simulink model "c00006M_harness"  (R2018a)
settings: Solver=FixedStepAuto  StartTime=0.0  StopTime=300  FixedStep=0.1  RelTol=1e-3
undefined symbols (not defined in the file): A1, hmax, PriorityTank, R1, R2, sigbuilder_block, TempThreshold
(part 3 of 66)

== system c00006M_harness/Eval150 ==
  In2 : Inport
  In3 : Inport  Port=2
  Constant1 : Constant
  Data Type Conversion1 : DataTypeConversion
  Data Type Conversion2 : DataTypeConversion
  Memory2 : Memory  InitialCondition=1
  Memory3 : Memory  InitialCondition=1
  MinMax : MinMax  Inputs=3
  MinMax2 : MinMax  Inputs=2
  MinMax3 : MinMax  Inputs=2
  ROOut2 : RelationalOperator  Operator===  OutDataTypeStr=boolean  RndMeth=Simplest
  ROOut3 : RelationalOperator  Operator===  OutDataTypeStr=boolean  RndMeth=Simplest
  Out1 : Outport
  wires:
  Data Type Conversion2/1 -> MinMax3/1
  Data Type Conversion1/1 -> MinMax2/1
  MinMax2/1 -> MinMax/2, Memory2/1
  Memory2/1 -> MinMax2/2
  Memory3/1 -> MinMax3/2
  ROOut2/1 -> Data Type Conversion1/1
  ROOut3/1 -> Data Type Conversion2/1
  MinMax3/1 -> Memory3/1, MinMax/3
  [out2] -> ROOut2/2
  In2/1 -> ROOut2/1
  In3/1 -> ROOut3/1
  [out3] -> ROOut3/2
  MinMax/1 -> Out1/1
  Constant1/1 -> MinMax/1

== system c00006M_harness/Eval151 ==
  In2 : Inport
  In3 : Inport  Port=2
  Constant1 : Constant
  Data Type Conversion1 : DataTypeConversion
  Data Type Conversion2 : DataTypeConversion
  Memory2 : Memory  InitialCondition=1
  Memory3 : Memory  InitialCondition=1
  MinMax : MinMax  Inputs=3
  MinMax2 : MinMax  Inputs=2
  MinMax3 : MinMax  Inputs=2
  ROOut2 : RelationalOperator  Operator===  OutDataTypeStr=boolean  RndMeth=Simplest
  ROOut3 : RelationalOperator  Operator===  OutDataTypeStr=boolean  RndMeth=Simplest
  Out1 : Outport
  wires:
  Data Type Conversion2/1 -> MinMax3/1
  Data Type Conversion1/1 -> MinMax2/1
  MinMax2/1 -> MinMax/2, Memory2/1
  Memory2/1 -> MinMax2/2
  Memory3/1 -> MinMax3/2
  ROOut2/1 -> Data Type Conversion1/1
  ROOut3/1 -> Data Type Conversion2/1
  MinMax3/1 -> Memory3/1, MinMax/3
  [out2] -> ROOut2/2
  In2/1 -> ROOut2/1
  In3/1 -> ROOut3/1
  [out3] -> ROOut3/2
  MinMax/1 -> Out1/1
  Constant1/1 -> MinMax/1

== system c00006M_harness/Eval152 ==
  In2 : Inport
  In3 : Inport  Port=2
  Constant1 : Constant
  Data Type Conversion1 : DataTypeConversion
  Data Type Conversion2 : DataTypeConversion
  Memory2 : Memory  InitialCondition=1
  Memory3 : Memory  InitialCondition=1
  MinMax : MinMax  Inputs=3
  MinMax2 : MinMax  Inputs=2
  MinMax3 : MinMax  Inputs=2
  ROOut2 : RelationalOperator  Operator===  OutDataTypeStr=boolean  RndMeth=Simplest
  ROOut3 : RelationalOperator  Operator===  OutDataTypeStr=boolean  RndMeth=Simplest
  Out1 : Outport
  wires:
  Data Type Conversion2/1 -> MinMax3/1
  Data Type Conversion1/1 -> MinMax2/1
  MinMax2/1 -> MinMax/2, Memory2/1
  Memory2/1 -> MinMax2/2
  Memory3/1 -> MinMax3/2
  ROOut2/1 -> Data Type Conversion1/1
  ROOut3/1 -> Data Type Conversion2/1
  MinMax3/1 -> Memory3/1, MinMax/3
  [out2] -> ROOut2/2
  In2/1 -> ROOut2/1
  In3/1 -> ROOut3/1
  [out3] -> ROOut3/2
  MinMax/1 -> Out1/1
  Constant1/1 -> MinMax/1

== system c00006M_harness/Eval153 ==
  In2 : Inport
  In3 : Inport  Port=2
  Constant1 : Constant
  Data Type Conversion1 : DataTypeConversion
  Data Type Conversion2 : DataTypeConversion
  Memory2 : Memory  InitialCondition=1
  Memory3 : Memory  InitialCondition=1
  MinMax : MinMax  Inputs=3
  MinMax2 : MinMax  Inputs=2
  MinMax3 : MinMax  Inputs=2
  ROOut2 : RelationalOperator  Operator===  OutDataTypeStr=boolean  RndMeth=Simplest
  ROOut3 : RelationalOperator  Operator===  OutDataTypeStr=boolean  RndMeth=Simplest
  Out1 : Outport
  wires:
  Data Type Conversion2/1 -> MinMax3/1
  Data Type Conversion1/1 -> MinMax2/1
  MinMax2/1 -> MinMax/2, Memory2/1
  Memory2/1 -> MinMax2/2
  Memory3/1 -> MinMax3/2
  ROOut2/1 -> Data Type Conversion1/1
  ROOut3/1 -> Data Type Conversion2/1
  MinMax3/1 -> Memory3/1, MinMax/3
  [out2] -> ROOut2/2
  In2/1 -> ROOut2/1
  In3/1 -> ROOut3/1
  [out3] -> ROOut3/2
  MinMax/1 -> Out1/1
  Constant1/1 -> MinMax/1

== system c00006M_harness/Eval154 ==
  In2 : Inport
  In3 : Inport  Port=2
  Constant1 : Constant
  Data Type Conversion1 : DataTypeConversion
  Data Type Conversion2 : DataTypeConversion
  Memory2 : Memory  InitialCondition=1
  Memory3 : Memory  InitialCondition=1
  MinMax : MinMax  Inputs=3
  MinMax2 : MinMax  Inputs=2
  MinMax3 : MinMax  Inputs=2
  ROOut2 : RelationalOperator  Operator===  OutDataTypeStr=boolean  RndMeth=Simplest
  ROOut3 : RelationalOperator  Operator===  OutDataTypeStr=boolean  RndMeth=Simplest
  Out1 : Outport
  wires:
  Data Type Conversion2/1 -> MinMax3/1
  Data Type Conversion1/1 -> MinMax2/1
  MinMax2/1 -> MinMax/2, Memory2/1
  Memory2/1 -> MinMax2/2
  Memory3/1 -> MinMax3/2
  ROOut2/1 -> Data Type Conversion1/1
  ROOut3/1 -> Data Type Conversion2/1
  MinMax3/1 -> Memory3/1, MinMax/3
  [out2] -> ROOut2/2
  In2/1 -> ROOut2/1
  In3/1 -> ROOut3/1
  [out3] -> ROOut3/2
  MinMax/1 -> Out1/1
  Constant1/1 -> MinMax/1

== system c00006M_harness/Eval155 ==
  In2 : Inport
  In3 : Inport  Port=2
  Constant1 : Constant
  Data Type Conversion1 : DataTypeConversion
  Data Type Conversion2 : DataTypeConversion
  Memory2 : Memory  InitialCondition=1
  Memory3 : Memory  InitialCondition=1
  MinMax : MinMax  Inputs=3
  MinMax2 : MinMax  Inputs=2
  MinMax3 : MinMax  Inputs=2
  ROOut2 : RelationalOperator  Operator===  OutDataTypeStr=boolean  RndMeth=Simplest
  ROOut3 : RelationalOperator  Operator===  OutDataTypeStr=boolean  RndMeth=Simplest
  Out1 : Outport
  wires:
  Data Type Conversion2/1 -> MinMax3/1
  Data Type Conversion1/1 -> MinMax2/1
  MinMax2/1 -> MinMax/2, Memory2/1
  Memory2/1 -> MinMax2/2
  Memory3/1 -> MinMax3/2
  ROOut2/1 -> Data Type Conversion1/1
  ROOut3/1 -> Data Type Conversion2/1
  MinMax3/1 -> Memory3/1, MinMax/3
  [out2] -> ROOut2/2
  In2/1 -> ROOut2/1
  In3/1 -> ROOut3/1
  [out3] -> ROOut3/2
  MinMax/1 -> Out1/1
  Constant1/1 -> MinMax/1

== system c00006M_harness/Eval156 ==
  In2 : Inport
  In3 : Inport  Port=2
  Constant1 : Constant
  Data Type Conversion1 : DataTypeConversion
  Data Type Conversion2 : DataTypeConversion
  Memory2 : Memory  InitialCondition=1
  Memory3 : Memory  InitialCondition=1
  MinMax : MinMax  Inputs=3
  MinMax2 : MinMax  Inputs=2
  MinMax3 : MinMax  Inputs=2
  ROOut2 : RelationalOperator  Operator===  OutDataTypeStr=boolean  RndMeth=Simplest
  ROOut3 : RelationalOperator  Operator===  OutDataTypeStr=boolean  RndMeth=Simplest
  Out1 : Outport
  wires:
  Data Type Conversion2/1 -> MinMax3/1
  Data Type Conversion1/1 -> MinMax2/1
  MinMax2/1 -> MinMax/2, Memory2/1
  Memory2/1 -> MinMax2/2
  Memory3/1 -> MinMax3/2
  ROOut2/1 -> Data Type Conversion1/1
  ROOut3/1 -> Data Type Conversion2/1
  MinMax3/1 -> Memory3/1, MinMax/3
  [out2] -> ROOut2/2
  In2/1 -> ROOut2/1
  In3/1 -> ROOut3/1
  [out3] -> ROOut3/2
  MinMax/1 -> Out1/1
  Constant1/1 -> MinMax/1

== system c00006M_harness/Eval157 ==
  In2 : Inport
  In3 : Inport  Port=2
  Constant1 : Constant
  Data Type Conversion1 : DataTypeConversion
  Data Type Conversion2 : DataTypeConversion
  Memory2 : Memory  InitialCondition=1
  Memory3 : Memory  InitialCondition=1
  MinMax : MinMax  Inputs=3
  MinMax2 : MinMax  Inputs=2
  MinMax3 : MinMax  Inputs=2
  ROOut2 : RelationalOperator  Operator===  OutDataTypeStr=boolean  RndMeth=Simplest
  ROOut3 : RelationalOperator  Operator===  OutDataTypeStr=boolean  RndMeth=Simplest
  Out1 : Outport
  wires:
  Data Type Conversion2/1 -> MinMax3/1
  Data Type Conversion1/1 -> MinMax2/1
  MinMax2/1 -> MinMax/2, Memory2/1
  Memory2/1 -> MinMax2/2
  Memory3/1 -> MinMax3/2
  ROOut2/1 -> Data Type Conversion1/1
  ROOut3/1 -> Data Type Conversion2/1
  MinMax3/1 -> Memory3/1, MinMax/3
  [out2] -> ROOut2/2
  In2/1 -> ROOut2/1
  In3/1 -> ROOut3/1
  [out3] -> ROOut3/2
  MinMax/1 -> Out1/1
  Constant1/1 -> MinMax/1

== system c00006M_harness/Eval158 ==
  In2 : Inport
  In3 : Inport  Port=2
  Constant1 : Constant
  Data Type Conversion1 : DataTypeConversion
  Data Type Conversion2 : DataTypeConversion
  Memory2 : Memory  InitialCondition=1
  Memory3 : Memory  InitialCondition=1
  MinMax : MinMax  Inputs=3
  MinMax2 : MinMax  Inputs=2
  MinMax3 : MinMax  Inputs=2
  ROOut2 : RelationalOperator  Operator===  OutDataTypeStr=boolean  RndMeth=Simplest
  ROOut3 : RelationalOperator  Operator===  OutDataTypeStr=boolean  RndMeth=Simplest
  Out1 : Outport
  wires:
  Data Type Conversion2/1 -> MinMax3/1
  Data Type Conversion1/1 -> MinMax2/1
  MinMax2/1 -> MinMax/2, Memory2/1
  Memory2/1 -> MinMax2/2
  Memory3/1 -> MinMax3/2
  ROOut2/1 -> Data Type Conversion1/1
  ROOut3/1 -> Data Type Conversion2/1
  MinMax3/1 -> Memory3/1, MinMax/3
  [out2] -> ROOut2/2
  In2/1 -> ROOut2/1
  In3/1 -> ROOut3/1
  [out3] -> ROOut3/2
  MinMax/1 -> Out1/1
  Constant1/1 -> MinMax/1

== system c00006M_harness/Eval159 ==
  In2 : Inport
  In3 : Inport  Port=2
  Constant1 : Constant
  Data Type Conversion1 : DataTypeConversion
  Data Type Conversion2 : DataTypeConversion
  Memory2 : Memory  InitialCondition=1
  Memory3 : Memory  InitialCondition=1
  MinMax : MinMax  Inputs=3
  MinMax2 : MinMax  Inputs=2
  MinMax3 : MinMax  Inputs=2
  ROOut2 : RelationalOperator  Operator===  OutDataTypeStr=boolean  RndMeth=Simplest
  ROOut3 : RelationalOperator  Operator===  OutDataTypeStr=boolean  RndMeth=Simplest
  Out1 : Outport
  wires:
  Data Type Conversion2/1 -> MinMax3/1
  Data Type Conversion1/1 -> MinMax2/1
  MinMax2/1 -> MinMax/2, Memory2/1
  Memory2/1 -> MinMax2/2
  Memory3/1 -> MinMax3/2
  ROOut2/1 -> Data Type Conversion1/1
  ROOut3/1 -> Data Type Conversion2/1
  MinMax3/1 -> Memory3/1, MinMax/3
  [out2] -> ROOut2/2
  In2/1 -> ROOut2/1
  In3/1 -> ROOut3/1
  [out3] -> ROOut3/2
  MinMax/1 -> Out1/1
  Constant1/1 -> MinMax/1

== system c00006M_harness/Eval160 ==
  In2 : Inport
  In3 : Inport  Port=2
  Constant1 : Constant
  Data Type Conversion1 : DataTypeConversion
  Data Type Conversion2 : DataTypeConversion
  Memory2 : Memory  InitialCondition=1
  Memory3 : Memory  InitialCondition=1
  MinMax : MinMax  Inputs=3
  MinMax2 : MinMax  Inputs=2
  MinMax3 : MinMax  Inputs=2
  ROOut2 : RelationalOperator  Operator===  OutDataTypeStr=boolean  RndMeth=Simplest
  ROOut3 : RelationalOperator  Operator===  OutDataTypeStr=boolean  RndMeth=Simplest
  Out1 : Outport
  wires:
  Data Type Conversion2/1 -> MinMax3/1
  Data Type Conversion1/1 -> MinMax2/1
  MinMax2/1 -> MinMax/2, Memory2/1
  Memory2/1 -> MinMax2/2
  Memory3/1 -> MinMax3/2
  ROOut2/1 -> Data Type Conversion1/1
  ROOut3/1 -> Data Type Conversion2/1
  MinMax3/1 -> Memory3/1, MinMax/3
  [out2] -> ROOut2/2
  In2/1 -> ROOut2/1
  In3/1 -> ROOut3/1
  [out3] -> ROOut3/2
  MinMax/1 -> Out1/1
  Constant1/1 -> MinMax/1

== system c00006M_harness/Eval161 ==
  In2 : Inport
  In3 : Inport  Port=2
  Constant1 : Constant
  Data Type Conversion1 : DataTypeConversion
  Data Type Conversion2 : DataTypeConversion
  Memory2 : Memory  InitialCondition=1
  Memory3 : Memory  InitialCondition=1
  MinMax : MinMax  Inputs=3
  MinMax2 : MinMax  Inputs=2
  MinMax3 : MinMax  Inputs=2
  ROOut2 : RelationalOperator  Operator===  OutDataTypeStr=boolean  RndMeth=Simplest
  ROOut3 : RelationalOperator  Operator===  OutDataTypeStr=boolean  RndMeth=Simplest
  Out1 : Outport
  wires:
  Data Type Conversion2/1 -> MinMax3/1
  Data Type Conversion1/1 -> MinMax2/1
  MinMax2/1 -> MinMax/2, Memory2/1
  Memory2/1 -> MinMax2/2
  Memory3/1 -> MinMax3/2
  ROOut2/1 -> Data Type Conversion1/1
  ROOut3/1 -> Data Type Conversion2/1
  MinMax3/1 -> Memory3/1, MinMax/3
  [out2] -> ROOut2/2
  In2/1 -> ROOut2/1
  In3/1 -> ROOut3/1
  [out3] -> ROOut3/2
  MinMax/1 -> Out1/1
  Constant1/1 -> MinMax/1

== system c00006M_harness/Eval162 ==
  In2 : Inport
  In3 : Inport  Port=2
  Constant1 : Constant
  Data Type Conversion1 : DataTypeConversion
  Data Type Conversion2 : DataTypeConversion
  Memory2 : Memory  InitialCondition=1
  Memory3 : Memory  InitialCondition=1
  MinMax : MinMax  Inputs=3
  MinMax2 : MinMax  Inputs=2
  MinMax3 : MinMax  Inputs=2
  ROOut2 : RelationalOperator  Operator===  OutDataTypeStr=boolean  RndMeth=Simplest
  ROOut3 : RelationalOperator  Operator===  OutDataTypeStr=boolean  RndMeth=Simplest
  Out1 : Outport
  wires:
  Data Type Conversion2/1 -> MinMax3/1
  Data Type Conversion1/1 -> MinMax2/1
  MinMax2/1 -> MinMax/2, Memory2/1
  Memory2/1 -> MinMax2/2
  Memory3/1 -> MinMax3/2
  ROOut2/1 -> Data Type Conversion1/1
  ROOut3/1 -> Data Type Conversion2/1
  MinMax3/1 -> Memory3/1, MinMax/3
  [out2] -> ROOut2/2
  In2/1 -> ROOut2/1
  In3/1 -> ROOut3/1
  [out3] -> ROOut3/2
  MinMax/1 -> Out1/1
  Constant1/1 -> MinMax/1

== system c00006M_harness/Eval163 ==
  In2 : Inport
  In3 : Inport  Port=2
  Constant1 : Constant
  Data Type Conversion1 : DataTypeConversion
  Data Type Conversion2 : DataTypeConversion
  Memory2 : Memory  InitialCondition=1
  Memory3 : Memory  InitialCondition=1
  MinMax : MinMax  Inputs=3
  MinMax2 : MinMax  Inputs=2
  MinMax3 : MinMax  Inputs=2
  ROOut2 : RelationalOperator  Operator===  OutDataTypeStr=boolean  RndMeth=Simplest
  ROOut3 : RelationalOperator  Operator===  OutDataTypeStr=boolean  RndMeth=Simplest
  Out1 : Outport
  wires:
  Data Type Conversion2/1 -> MinMax3/1
  Data Type Conversion1/1 -> MinMax2/1
  MinMax2/1 -> MinMax/2, Memory2/1
  Memory2/1 -> MinMax2/2
  Memory3/1 -> MinMax3/2
  ROOut2/1 -> Data Type Conversion1/1
  ROOut3/1 -> Data Type Conversion2/1
  MinMax3/1 -> Memory3/1, MinMax/3
  [out2] -> ROOut2/2
  In2/1 -> ROOut2/1
  In3/1 -> ROOut3/1
  [out3] -> ROOut3/2
  MinMax/1 -> Out1/1
  Constant1/1 -> MinMax/1

== system c00006M_harness/Eval164 ==
  In2 : Inport
  In3 : Inport  Port=2
  Constant1 : Constant
  Data Type Conversion1 : DataTypeConversion
  Data Type Conversion2 : DataTypeConversion
  Memory2 : Memory  InitialCondition=1
  Memory3 : Memory  InitialCondition=1
  MinMax : MinMax  Inputs=3
  MinMax2 : MinMax  Inputs=2
  MinMax3 : MinMax  Inputs=2
  ROOut2 : RelationalOperator  Operator===  OutDataTypeStr=boolean  RndMeth=Simplest
  ROOut3 : RelationalOperator  Operator===  OutDataTypeStr=boolean  RndMeth=Simplest
  Out1 : Outport
  wires:
  Data Type Conversion2/1 -> MinMax3/1
  Data Type Conversion1/1 -> MinMax2/1
  MinMax2/1 -> MinMax/2, Memory2/1
  Memory2/1 -> MinMax2/2
  Memory3/1 -> MinMax3/2
  ROOut2/1 -> Data Type Conversion1/1
  ROOut3/1 -> Data Type Conversion2/1
  MinMax3/1 -> Memory3/1, MinMax/3
  [out2] -> ROOut2/2
  In2/1 -> ROOut2/1
  In3/1 -> ROOut3/1
  [out3] -> ROOut3/2
  MinMax/1 -> Out1/1
  Constant1/1 -> MinMax/1

== system c00006M_harness/Eval165 ==
  In2 : Inport
  In3 : Inport  Port=2
  Constant1 : Constant
  Data Type Conversion1 : DataTypeConversion
  Data Type Conversion2 : DataTypeConversion
  Memory2 : Memory  InitialCondition=1
  Memory3 : Memory  InitialCondition=1
  MinMax : MinMax  Inputs=3
  MinMax2 : MinMax  Inputs=2
  MinMax3 : MinMax  Inputs=2
  ROOut2 : RelationalOperator  Operator===  OutDataTypeStr=boolean  RndMeth=Simplest
  ROOut3 : RelationalOperator  Operator===  OutDataTypeStr=boolean  RndMeth=Simplest
  Out1 : Outport
  wires:
  Data Type Conversion2/1 -> MinMax3/1
  Data Type Conversion1/1 -> MinMax2/1
  MinMax2/1 -> MinMax/2, Memory2/1
  Memory2/1 -> MinMax2/2
  Memory3/1 -> MinMax3/2
  ROOut2/1 -> Data Type Conversion1/1
  ROOut3/1 -> Data Type Conversion2/1
  MinMax3/1 -> Memory3/1, MinMax/3
  [out2] -> ROOut2/2
  In2/1 -> ROOut2/1
  In3/1 -> ROOut3/1
  [out3] -> ROOut3/2
  MinMax/1 -> Out1/1
  Constant1/1 -> MinMax/1

== system c00006M_harness/Eval166 ==
  In2 : Inport
  In3 : Inport  Port=2
  Constant1 : Constant
  Data Type Conversion1 : DataTypeConversion
  Data Type Conversion2 : DataTypeConversion
  Memory2 : Memory  InitialCondition=1
  Memory3 : Memory  InitialCondition=1
  MinMax : MinMax  Inputs=3
  MinMax2 : MinMax  Inputs=2
  MinMax3 : MinMax  Inputs=2
  ROOut2 : RelationalOperator  Operator===  OutDataTypeStr=boolean  RndMeth=Simplest
  ROOut3 : RelationalOperator  Operator===  OutDataTypeStr=boolean  RndMeth=Simplest
  Out1 : Outport
  wires:
  Data Type Conversion2/1 -> MinMax3/1
  Data Type Conversion1/1 -> MinMax2/1
  MinMax2/1 -> MinMax/2, Memory2/1
  Memory2/1 -> MinMax2/2
  Memory3/1 -> MinMax3/2
  ROOut2/1 -> Data Type Conversion1/1
  ROOut3/1 -> Data Type Conversion2/1
  MinMax3/1 -> Memory3/1, MinMax/3
  [out2] -> ROOut2/2
  In2/1 -> ROOut2/1
  In3/1 -> ROOut3/1
  [out3] -> ROOut3/2
  MinMax/1 -> Out1/1
  Constant1/1 -> MinMax/1

== system c00006M_harness/Eval167 ==
  In2 : Inport
  In3 : Inport  Port=2
  Constant1 : Constant
  Data Type Conversion1 : DataTypeConversion
  Data Type Conversion2 : DataTypeConversion
  Memory2 : Memory  InitialCondition=1
  Memory3 : Memory  InitialCondition=1
  MinMax : MinMax  Inputs=3
  MinMax2 : MinMax  Inputs=2
  MinMax3 : MinMax  Inputs=2
  ROOut2 : RelationalOperator  Operator===  OutDataTypeStr=boolean  RndMeth=Simplest
  ROOut3 : RelationalOperator  Operator===  OutDataTypeStr=boolean  RndMeth=Simplest
  Out1 : Outport
  wires:
  Data Type Conversion2/1 -> MinMax3/1
  Data Type Conversion1/1 -> MinMax2/1
  MinMax2/1 -> MinMax/2, Memory2/1
  Memory2/1 -> MinMax2/2
  Memory3/1 -> MinMax3/2
  ROOut2/1 -> Data Type Conversion1/1
  ROOut3/1 -> Data Type Conversion2/1
  MinMax3/1 -> Memory3/1, MinMax/3
  [out2] -> ROOut2/2
  In2/1 -> ROOut2/1
  In3/1 -> ROOut3/1
  [out3] -> ROOut3/2
  MinMax/1 -> Out1/1
  Constant1/1 -> MinMax/1

== system c00006M_harness/Eval168 ==
  In2 : Inport
  In3 : Inport  Port=2
  Constant1 : Constant
  Data Type Conversion1 : DataTypeConversion
  Data Type Conversion2 : DataTypeConversion
  Memory2 : Memory  InitialCondition=1
  Memory3 : Memory  InitialCondition=1
  MinMax : MinMax  Inputs=3
  MinMax2 : MinMax  Inputs=2
  MinMax3 : MinMax  Inputs=2
  ROOut2 : RelationalOperator  Operator===  OutDataTypeStr=boolean  RndMeth=Simplest
  ROOut3 : RelationalOperator  Operator===  OutDataTypeStr=boolean  RndMeth=Simplest
  Out1 : Outport
  wires:
  Data Type Conversion2/1 -> MinMax3/1
  Data Type Conversion1/1 -> MinMax2/1
  MinMax2/1 -> MinMax/2, Memory2/1
  Memory2/1 -> MinMax2/2
  Memory3/1 -> MinMax3/2
  ROOut2/1 -> Data Type Conversion1/1
  ROOut3/1 -> Data Type Conversion2/1
  MinMax3/1 -> Memory3/1, MinMax/3
  [out2] -> ROOut2/2
  In2/1 -> ROOut2/1
  In3/1 -> ROOut3/1
  [out3] -> ROOut3/2
  MinMax/1 -> Out1/1
  Constant1/1 -> MinMax/1

== system c00006M_harness/Eval169 ==
  In2 : Inport
  In3 : Inport  Port=2
  Constant1 : Constant
  Data Type Conversion1 : DataTypeConversion
  Data Type Conversion2 : DataTypeConversion
  Memory2 : Memory  InitialCondition=1
  Memory3 : Memory  InitialCondition=1
  MinMax : MinMax  Inputs=3
  MinMax2 : MinMax  Inputs=2
  MinMax3 : MinMax  Inputs=2
  ROOut2 : RelationalOperator  Operator===  OutDataTypeStr=boolean  RndMeth=Simplest
  ROOut3 : RelationalOperator  Operator===  OutDataTypeStr=boolean  RndMeth=Simplest
  Out1 : Outport
  wires:
  Data Type Conversion2/1 -> MinMax3/1
  Data Type Conversion1/1 -> MinMax2/1
  MinMax2/1 -> MinMax/2, Memory2/1
  Memory2/1 -> MinMax2/2
  Memory3/1 -> MinMax3/2
  ROOut2/1 -> Data Type Conversion1/1
  ROOut3/1 -> Data Type Conversion2/1
  MinMax3/1 -> Memory3/1, MinMax/3
  [out2] -> ROOut2/2
  In2/1 -> ROOut2/1
  In3/1 -> ROOut3/1
  [out3] -> ROOut3/2
  MinMax/1 -> Out1/1
  Constant1/1 -> MinMax/1

== system c00006M_harness/Eval170 ==
  In2 : Inport
  In3 : Inport  Port=2
  Constant1 : Constant
  Data Type Conversion1 : DataTypeConversion
  Data Type Conversion2 : DataTypeConversion
  Memory2 : Memory  InitialCondition=1
  Memory3 : Memory  InitialCondition=1
  MinMax : MinMax  Inputs=3
  MinMax2 : MinMax  Inputs=2
  MinMax3 : MinMax  Inputs=2
  ROOut2 : RelationalOperator  Operator===  OutDataTypeStr=boolean  RndMeth=Simplest
  ROOut3 : RelationalOperator  Operator===  OutDataTypeStr=boolean  RndMeth=Simplest
  Out1 : Outport
  wires:
  Data Type Conversion2/1 -> MinMax3/1
  Data Type Conversion1/1 -> MinMax2/1
  MinMax2/1 -> MinMax/2, Memory2/1
  Memory2/1 -> MinMax2/2
  Memory3/1 -> MinMax3/2
  ROOut2/1 -> Data Type Conversion1/1
  ROOut3/1 -> Data Type Conversion2/1
  MinMax3/1 -> Memory3/1, MinMax/3
  [out2] -> ROOut2/2
  In2/1 -> ROOut2/1
  In3/1 -> ROOut3/1
  [out3] -> ROOut3/2
  MinMax/1 -> Out1/1
  Constant1/1 -> MinMax/1

== system c00006M_harness/Eval171 ==
  In2 : Inport
  In3 : Inport  Port=2
  Constant1 : Constant
  Data Type Conversion1 : DataTypeConversion
  Data Type Conversion2 : DataTypeConversion
  Memory2 : Memory  InitialCondition=1
  Memory3 : Memory  InitialCondition=1
  MinMax : MinMax  Inputs=3
  MinMax2 : MinMax  Inputs=2
  MinMax3 : MinMax  Inputs=2
  ROOut2 : RelationalOperator  Operator===  OutDataTypeStr=boolean  RndMeth=Simplest
  ROOut3 : RelationalOperator  Operator===  OutDataTypeStr=boolean  RndMeth=Simplest
  Out1 : Outport
  wires:
  Data Type Conversion2/1 -> MinMax3/1
  Data Type Conversion1/1 -> MinMax2/1
  MinMax2/1 -> MinMax/2, Memory2/1
  Memory2/1 -> MinMax2/2
  Memory3/1 -> MinMax3/2
  ROOut2/1 -> Data Type Conversion1/1
  ROOut3/1 -> Data Type Conversion2/1
  MinMax3/1 -> Memory3/1, MinMax/3
  [out2] -> ROOut2/2
  In2/1 -> ROOut2/1
  In3/1 -> ROOut3/1
  [out3] -> ROOut3/2
  MinMax/1 -> Out1/1
  Constant1/1 -> MinMax/1

== system c00006M_harness/Eval172 ==
  In2 : Inport
  In3 : Inport  Port=2
  Constant1 : Constant
  Data Type Conversion1 : DataTypeConversion
  Data Type Conversion2 : DataTypeConversion
  Memory2 : Memory  InitialCondition=1
  Memory3 : Memory  InitialCondition=1
  MinMax : MinMax  Inputs=3
  MinMax2 : MinMax  Inputs=2
  MinMax3 : MinMax  Inputs=2
  ROOut2 : RelationalOperator  Operator===  OutDataTypeStr=boolean  RndMeth=Simplest
  ROOut3 : RelationalOperator  Operator===  OutDataTypeStr=boolean  RndMeth=Simplest
  Out1 : Outport
  wires:
  Data Type Conversion2/1 -> MinMax3/1
  Data Type Conversion1/1 -> MinMax2/1
  MinMax2/1 -> MinMax/2, Memory2/1
  Memory2/1 -> MinMax2/2
  Memory3/1 -> MinMax3/2
  ROOut2/1 -> Data Type Conversion1/1
  ROOut3/1 -> Data Type Conversion2/1
  MinMax3/1 -> Memory3/1, MinMax/3
  [out2] -> ROOut2/2
  In2/1 -> ROOut2/1
  In3/1 -> ROOut3/1
  [out3] -> ROOut3/2
  MinMax/1 -> Out1/1
  Constant1/1 -> MinMax/1

== system c00006M_harness/Eval173 ==
  In2 : Inport
  In3 : Inport  Port=2
  Constant1 : Constant
  Data Type Conversion1 : DataTypeConversion
  Data Type Conversion2 : DataTypeConversion
  Memory2 : Memory  InitialCondition=1
  Memory3 : Memory  InitialCondition=1
  MinMax : MinMax  Inputs=3
  MinMax2 : MinMax  Inputs=2
  MinMax3 : MinMax  Inputs=2
  ROOut2 : RelationalOperator  Operator===  OutDataTypeStr=boolean  RndMeth=Simplest
  ROOut3 : RelationalOperator  Operator===  OutDataTypeStr=boolean  RndMeth=Simplest
  Out1 : Outport
  wires:
  Data Type Conversion2/1 -> MinMax3/1
  Data Type Conversion1/1 -> MinMax2/1
  MinMax2/1 -> MinMax/2, Memory2/1
  Memory2/1 -> MinMax2/2
  Memory3/1 -> MinMax3/2
  ROOut2/1 -> Data Type Conversion1/1
  ROOut3/1 -> Data Type Conversion2/1
  MinMax3/1 -> Memory3/1, MinMax/3
  [out2] -> ROOut2/2
  In2/1 -> ROOut2/1
  In3/1 -> ROOut3/1
  [out3] -> ROOut3/2
  MinMax/1 -> Out1/1
  Constant1/1 -> MinMax/1

== system c00006M_harness/Eval174 ==
  In2 : Inport
  In3 : Inport  Port=2
  Constant1 : Constant
  Data Type Conversion1 : DataTypeConversion
  Data Type Conversion2 : DataTypeConversion
  Memory2 : Memory  InitialCondition=1
  Memory3 : Memory  InitialCondition=1
  MinMax : MinMax  Inputs=3
  MinMax2 : MinMax  Inputs=2
  MinMax3 : MinMax  Inputs=2
  ROOut2 : RelationalOperator  Operator===  OutDataTypeStr=boolean  RndMeth=Simplest
  ROOut3 : RelationalOperator  Operator===  OutDataTypeStr=boolean  RndMeth=Simplest
  Out1 : Outport
  wires:
  Data Type Conversion2/1 -> MinMax3/1
  Data Type Conversion1/1 -> MinMax2/1
  MinMax2/1 -> MinMax/2, Memory2/1
  Memory2/1 -> MinMax2/2
  Memory3/1 -> MinMax3/2
  ROOut2/1 -> Data Type Conversion1/1
  ROOut3/1 -> Data Type Conversion2/1
  MinMax3/1 -> Memory3/1, MinMax/3
  [out2] -> ROOut2/2
  In2/1 -> ROOut2/1
  In3/1 -> ROOut3/1
  [out3] -> ROOut3/2
  MinMax/1 -> Out1/1
  Constant1/1 -> MinMax/1

== system c00006M_harness/Eval175 ==
  In2 : Inport
  In3 : Inport  Port=2
  Constant1 : Constant
  Data Type Conversion1 : DataTypeConversion
  Data Type Conversion2 : DataTypeConversion
  Memory2 : Memory  InitialCondition=1
  Memory3 : Memory  InitialCondition=1
  MinMax : MinMax  Inputs=3
  MinMax2 : MinMax  Inputs=2
  MinMax3 : MinMax  Inputs=2
  ROOut2 : RelationalOperator  Operator===  OutDataTypeStr=boolean  RndMeth=Simplest
  ROOut3 : RelationalOperator  Operator===  OutDataTypeStr=boolean  RndMeth=Simplest
  Out1 : Outport
  wires:
  Data Type Conversion2/1 -> MinMax3/1
  Data Type Conversion1/1 -> MinMax2/1
  MinMax2/1 -> MinMax/2, Memory2/1
  Memory2/1 -> MinMax2/2
  Memory3/1 -> MinMax3/2
  ROOut2/1 -> Data Type Conversion1/1
  ROOut3/1 -> Data Type Conversion2/1
  MinMax3/1 -> Memory3/1, MinMax/3
  [out2] -> ROOut2/2
  In2/1 -> ROOut2/1
  In3/1 -> ROOut3/1
  [out3] -> ROOut3/2
  MinMax/1 -> Out1/1
  Constant1/1 -> MinMax/1

== system c00006M_harness/Eval176 ==
  In2 : Inport
  In3 : Inport  Port=2
  Constant1 : Constant
  Data Type Conversion1 : DataTypeConversion
  Data Type Conversion2 : DataTypeConversion
  Memory2 : Memory  InitialCondition=1
  Memory3 : Memory  InitialCondition=1
  MinMax : MinMax  Inputs=3
  MinMax2 : MinMax  Inputs=2
  MinMax3 : MinMax  Inputs=2
  ROOut2 : RelationalOperator  Operator===  OutDataTypeStr=boolean  RndMeth=Simplest
  ROOut3 : RelationalOperator  Operator===  OutDataTypeStr=boolean  RndMeth=Simplest
  Out1 : Outport
  wires:
  Data Type Conversion2/1 -> MinMax3/1
  Data Type Conversion1/1 -> MinMax2/1
  MinMax2/1 -> MinMax/2, Memory2/1
  Memory2/1 -> MinMax2/2
  Memory3/1 -> MinMax3/2
  ROOut2/1 -> Data Type Conversion1/1
  ROOut3/1 -> Data Type Conversion2/1
  MinMax3/1 -> Memory3/1, MinMax/3
  [out2] -> ROOut2/2
  In2/1 -> ROOut2/1
  In3/1 -> ROOut3/1
  [out3] -> ROOut3/2
  MinMax/1 -> Out1/1
  Constant1/1 -> MinMax/1

== system c00006M_harness/Eval177 ==
  In2 : Inport
  In3 : Inport  Port=2
  Constant1 : Constant
  Data Type Conversion1 : DataTypeConversion
  Data Type Conversion2 : DataTypeConversion
  Memory2 : Memory  InitialCondition=1
  Memory3 : Memory  InitialCondition=1
  MinMax : MinMax  Inputs=3
  MinMax2 : MinMax  Inputs=2
  MinMax3 : MinMax  Inputs=2
  ROOut2 : RelationalOperator  Operator===  OutDataTypeStr=boolean  RndMeth=Simplest
  ROOut3 : RelationalOperator  Operator===  OutDataTypeStr=boolean  RndMeth=Simplest
  Out1 : Outport
  wires:
  Data Type Conversion2/1 -> MinMax3/1
  Data Type Conversion1/1 -> MinMax2/1
  MinMax2/1 -> MinMax/2, Memory2/1
  Memory2/1 -> MinMax2/2
  Memory3/1 -> MinMax3/2
  ROOut2/1 -> Data Type Conversion1/1
  ROOut3/1 -> Data Type Conversion2/1
  MinMax3/1 -> Memory3/1, MinMax/3
  [out2] -> ROOut2/2
  In2/1 -> ROOut2/1
  In3/1 -> ROOut3/1
  [out3] -> ROOut3/2
  MinMax/1 -> Out1/1
  Constant1/1 -> MinMax/1

== system c00006M_harness/Eval178 ==
  In2 : Inport
  In3 : Inport  Port=2
  Constant1 : Constant
  Data Type Conversion1 : DataTypeConversion
  Data Type Conversion2 : DataTypeConversion
  Memory2 : Memory  InitialCondition=1
  Memory3 : Memory  InitialCondition=1
  MinMax : MinMax  Inputs=3
  MinMax2 : MinMax  Inputs=2
  MinMax3 : MinMax  Inputs=2
  ROOut2 : RelationalOperator  Operator===  OutDataTypeStr=boolean  RndMeth=Simplest
  ROOut3 : RelationalOperator  Operator===  OutDataTypeStr=boolean  RndMeth=Simplest
  Out1 : Outport
  wires:
  Data Type Conversion2/1 -> MinMax3/1
  Data Type Conversion1/1 -> MinMax2/1
  MinMax2/1 -> MinMax/2, Memory2/1
  Memory2/1 -> MinMax2/2
  Memory3/1 -> MinMax3/2
  ROOut2/1 -> Data Type Conversion1/1
  ROOut3/1 -> Data Type Conversion2/1
  MinMax3/1 -> Memory3/1, MinMax/3
  [out2] -> ROOut2/2
  In2/1 -> ROOut2/1
  In3/1 -> ROOut3/1
  [out3] -> ROOut3/2
  MinMax/1 -> Out1/1
  Constant1/1 -> MinMax/1

== system c00006M_harness/Eval179 ==
  In2 : Inport
  In3 : Inport  Port=2
  Constant1 : Constant
  Data Type Conversion1 : DataTypeConversion
  Data Type Conversion2 : DataTypeConversion
  Memory2 : Memory  InitialCondition=1
  Memory3 : Memory  InitialCondition=1
  MinMax : MinMax  Inputs=3
  MinMax2 : MinMax  Inputs=2
  MinMax3 : MinMax  Inputs=2
  ROOut2 : RelationalOperator  Operator===  OutDataTypeStr=boolean  RndMeth=Simplest
  ROOut3 : RelationalOperator  Operator===  OutDataTypeStr=boolean  RndMeth=Simplest
  Out1 : Outport
  wires:
  Data Type Conversion2/1 -> MinMax3/1
  Data Type Conversion1/1 -> MinMax2/1
  MinMax2/1 -> MinMax/2, Memory2/1
  Memory2/1 -> MinMax2/2
  Memory3/1 -> MinMax3/2
  ROOut2/1 -> Data Type Conversion1/1
  ROOut3/1 -> Data Type Conversion2/1
  MinMax3/1 -> Memory3/1, MinMax/3
  [out2] -> ROOut2/2
  In2/1 -> ROOut2/1
  In3/1 -> ROOut3/1
  [out3] -> ROOut3/2
  MinMax/1 -> Out1/1
  Constant1/1 -> MinMax/1

== system c00006M_harness/Eval180 ==
  In2 : Inport
  In3 : Inport  Port=2
  Constant1 : Constant
  Data Type Conversion1 : DataTypeConversion
  Data Type Conversion2 : DataTypeConversion
  Memory2 : Memory  InitialCondition=1
  Memory3 : Memory  InitialCondition=1
  MinMax : MinMax  Inputs=3
  MinMax2 : MinMax  Inputs=2
  MinMax3 : MinMax  Inputs=2
  ROOut2 : RelationalOperator  Operator===  OutDataTypeStr=boolean  RndMeth=Simplest
  ROOut3 : RelationalOperator  Operator===  OutDataTypeStr=boolean  RndMeth=Simplest
  Out1 : Outport
  wires:
  Data Type Conversion2/1 -> MinMax3/1
  Data Type Conversion1/1 -> MinMax2/1
  MinMax2/1 -> MinMax/2, Memory2/1
  Memory2/1 -> MinMax2/2
  Memory3/1 -> MinMax3/2
  ROOut2/1 -> Data Type Conversion1/1
  ROOut3/1 -> Data Type Conversion2/1
  MinMax3/1 -> Memory3/1, MinMax/3
  [out2] -> ROOut2/2
  In2/1 -> ROOut2/1
  In3/1 -> ROOut3/1
  [out3] -> ROOut3/2
  MinMax/1 -> Out1/1
  Constant1/1 -> MinMax/1

== system c00006M_harness/Eval181 ==
  In2 : Inport
  In3 : Inport  Port=2
  Constant1 : Constant
  Data Type Conversion1 : DataTypeConversion
  Data Type Conversion2 : DataTypeConversion
  Memory2 : Memory  InitialCondition=1
  Memory3 : Memory  InitialCondition=1
  MinMax : MinMax  Inputs=3
  MinMax2 : MinMax  Inputs=2
  MinMax3 : MinMax  Inputs=2
  ROOut2 : RelationalOperator  Operator===  OutDataTypeStr=boolean  RndMeth=Simplest
  ROOut3 : RelationalOperator  Operator===  OutDataTypeStr=boolean  RndMeth=Simplest
  Out1 : Outport
  wires:
  Data Type Conversion2/1 -> MinMax3/1
  Data Type Conversion1/1 -> MinMax2/1
  MinMax2/1 -> MinMax/2, Memory2/1
  Memory2/1 -> MinMax2/2
  Memory3/1 -> MinMax3/2
  ROOut2/1 -> Data Type Conversion1/1
  ROOut3/1 -> Data Type Conversion2/1
  MinMax3/1 -> Memory3/1, MinMax/3
  [out2] -> ROOut2/2
  In2/1 -> ROOut2/1
  In3/1 -> ROOut3/1
  [out3] -> ROOut3/2
  MinMax/1 -> Out1/1
  Constant1/1 -> MinMax/1

== system c00006M_harness/Eval182 ==
  In2 : Inport
  In3 : Inport  Port=2
  Constant1 : Constant
  Data Type Conversion1 : DataTypeConversion
  Data Type Conversion2 : DataTypeConversion
  Memory2 : Memory  InitialCondition=1
  Memory3 : Memory  InitialCondition=1
  MinMax : MinMax  Inputs=3
  MinMax2 : MinMax  Inputs=2
  MinMax3 : MinMax  Inputs=2
  ROOut2 : RelationalOperator  Operator===  OutDataTypeStr=boolean  RndMeth=Simplest
  ROOut3 : RelationalOperator  Operator===  OutDataTypeStr=boolean  RndMeth=Simplest
  Out1 : Outport
  wires:
  Data Type Conversion2/1 -> MinMax3/1
  Data Type Conversion1/1 -> MinMax2/1
  MinMax2/1 -> MinMax/2, Memory2/1
  Memory2/1 -> MinMax2/2
  Memory3/1 -> MinMax3/2
  ROOut2/1 -> Data Type Conversion1/1
  ROOut3/1 -> Data Type Conversion2/1
  MinMax3/1 -> Memory3/1, MinMax/3
  [out2] -> ROOut2/2
  In2/1 -> ROOut2/1
  In3/1 -> ROOut3/1
  [out3] -> ROOut3/2
  MinMax/1 -> Out1/1
  Constant1/1 -> MinMax/1

== system c00006M_harness/Eval183 ==
  In2 : Inport
  In3 : Inport  Port=2
  Constant1 : Constant
  Data Type Conversion1 : DataTypeConversion
  Data Type Conversion2 : DataTypeConversion
  Memory2 : Memory  InitialCondition=1
  Memory3 : Memory  InitialCondition=1
  MinMax : MinMax  Inputs=3
  MinMax2 : MinMax  Inputs=2
  MinMax3 : MinMax  Inputs=2
  ROOut2 : RelationalOperator  Operator===  OutDataTypeStr=boolean  RndMeth=Simplest
  ROOut3 : RelationalOperator  Operator===  OutDataTypeStr=boolean  RndMeth=Simplest
  Out1 : Outport
  wires:
  Data Type Conversion2/1 -> MinMax3/1
  Data Type Conversion1/1 -> MinMax2/1
  MinMax2/1 -> MinMax/2, Memory2/1
  Memory2/1 -> MinMax2/2
  Memory3/1 -> MinMax3/2
  ROOut2/1 -> Data Type Conversion1/1
  ROOut3/1 -> Data Type Conversion2/1
  MinMax3/1 -> Memory3/1, MinMax/3
  [out2] -> ROOut2/2
  In2/1 -> ROOut2/1
  In3/1 -> ROOut3/1
  [out3] -> ROOut3/2
  MinMax/1 -> Out1/1
  Constant1/1 -> MinMax/1

== system c00006M_harness/Eval184 ==
  In2 : Inport
  In3 : Inport  Port=2
  Constant1 : Constant
  Data Type Conversion1 : DataTypeConversion
  Data Type Conversion2 : DataTypeConversion
  Memory2 : Memory  InitialCondition=1
  Memory3 : Memory  InitialCondition=1
  MinMax : MinMax  Inputs=3
  MinMax2 : MinMax  Inputs=2
  MinMax3 : MinMax  Inputs=2
  ROOut2 : RelationalOperator  Operator===  OutDataTypeStr=boolean  RndMeth=Simplest
  ROOut3 : RelationalOperator  Operator===  OutDataTypeStr=boolean  RndMeth=Simplest
  Out1 : Outport
  wires:
  Data Type Conversion2/1 -> MinMax3/1
  Data Type Conversion1/1 -> MinMax2/1
  MinMax2/1 -> MinMax/2, Memory2/1
  Memory2/1 -> MinMax2/2
  Memory3/1 -> MinMax3/2
  ROOut2/1 -> Data Type Conversion1/1
  ROOut3/1 -> Data Type Conversion2/1
  MinMax3/1 -> Memory3/1, MinMax/3
  [out2] -> ROOut2/2
  In2/1 -> ROOut2/1
  In3/1 -> ROOut3/1
  [out3] -> ROOut3/2
  MinMax/1 -> Out1/1
  Constant1/1 -> MinMax/1

== system c00006M_harness/Eval185 ==
  In2 : Inport
  In3 : Inport  Port=2
  Constant1 : Constant
  Data Type Conversion1 : DataTypeConversion
  Data Type Conversion2 : DataTypeConversion
  Memory2 : Memory  InitialCondition=1
  Memory3 : Memory  InitialCondition=1
  MinMax : MinMax  Inputs=3
  MinMax2 : MinMax  Inputs=2
  MinMax3 : MinMax  Inputs=2
  ROOut2 : RelationalOperator  Operator===  OutDataTypeStr=boolean  RndMeth=Simplest
  ROOut3 : RelationalOperator  Operator===  OutDataTypeStr=boolean  RndMeth=Simplest
  Out1 : Outport
  wires:
  Data Type Conversion2/1 -> MinMax3/1
  Data Type Conversion1/1 -> MinMax2/1
  MinMax2/1 -> MinMax/2, Memory2/1
  Memory2/1 -> MinMax2/2
  Memory3/1 -> MinMax3/2
  ROOut2/1 -> Data Type Conversion1/1
  ROOut3/1 -> Data Type Conversion2/1
  MinMax3/1 -> Memory3/1, MinMax/3
  [out2] -> ROOut2/2
  In2/1 -> ROOut2/1
  In3/1 -> ROOut3/1
  [out3] -> ROOut3/2
  MinMax/1 -> Out1/1
  Constant1/1 -> MinMax/1

== system c00006M_harness/Eval186 ==
  In2 : Inport
  In3 : Inport  Port=2
  Constant1 : Constant
  Data Type Conversion1 : DataTypeConversion
  Data Type Conversion2 : DataTypeConversion
  Memory2 : Memory  InitialCondition=1
  Memory3 : Memory  InitialCondition=1
  MinMax : MinMax  Inputs=3
  MinMax2 : MinMax  Inputs=2
  MinMax3 : MinMax  Inputs=2
  ROOut2 : RelationalOperator  Operator===  OutDataTypeStr=boolean  RndMeth=Simplest
  ROOut3 : RelationalOperator  Operator===  OutDataTypeStr=boolean  RndMeth=Simplest
  Out1 : Outport
  wires:
  Data Type Conversion2/1 -> MinMax3/1
  Data Type Conversion1/1 -> MinMax2/1
  MinMax2/1 -> MinMax/2, Memory2/1
  Memory2/1 -> MinMax2/2
  Memory3/1 -> MinMax3/2
  ROOut2/1 -> Data Type Conversion1/1
  ROOut3/1 -> Data Type Conversion2/1
  MinMax3/1 -> Memory3/1, MinMax/3
  [out2] -> ROOut2/2
  In2/1 -> ROOut2/1
  In3/1 -> ROOut3/1
  [out3] -> ROOut3/2
  MinMax/1 -> Out1/1
  Constant1/1 -> MinMax/1

== system c00006M_harness/Eval187 ==
  In2 : Inport
  In3 : Inport  Port=2
  Constant1 : Constant
  Data Type Conversion1 : DataTypeConversion
  Data Type Conversion2 : DataTypeConversion
  Memory2 : Memory  InitialCondition=1
  Memory3 : Memory  InitialCondition=1
  MinMax : MinMax  Inputs=3
  MinMax2 : MinMax  Inputs=2
  MinMax3 : MinMax  Inputs=2
  ROOut2 : RelationalOperator  Operator===  OutDataTypeStr=boolean  RndMeth=Simplest
  ROOut3 : RelationalOperator  Operator===  OutDataTypeStr=boolean  RndMeth=Simplest
  Out1 : Outport
  wires:
  Data Type Conversion2/1 -> MinMax3/1
  Data Type Conversion1/1 -> MinMax2/1
  MinMax2/1 -> MinMax/2, Memory2/1
  Memory2/1 -> MinMax2/2
  Memory3/1 -> MinMax3/2
  ROOut2/1 -> Data Type Conversion1/1
  ROOut3/1 -> Data Type Conversion2/1
  MinMax3/1 -> Memory3/1, MinMax/3
  [out2] -> ROOut2/2
  In2/1 -> ROOut2/1
  In3/1 -> ROOut3/1
  [out3] -> ROOut3/2
  MinMax/1 -> Out1/1
  Constant1/1 -> MinMax/1

== system c00006M_harness/Eval188 ==
  In2 : Inport
  In3 : Inport  Port=2
  Constant1 : Constant
  Data Type Conversion1 : DataTypeConversion
  Data Type Conversion2 : DataTypeConversion
  Memory2 : Memory  InitialCondition=1
  Memory3 : Memory  InitialCondition=1
  MinMax : MinMax  Inputs=3
  MinMax2 : MinMax  Inputs=2
  MinMax3 : MinMax  Inputs=2
  ROOut2 : RelationalOperator  Operator===  OutDataTypeStr=boolean  RndMeth=Simplest
  ROOut3 : RelationalOperator  Operator===  OutDataTypeStr=boolean  RndMeth=Simplest
  Out1 : Outport
  wires:
  Data Type Conversion2/1 -> MinMax3/1
  Data Type Conversion1/1 -> MinMax2/1
  MinMax2/1 -> MinMax/2, Memory2/1
  Memory2/1 -> MinMax2/2
  Memory3/1 -> MinMax3/2
  ROOut2/1 -> Data Type Conversion1/1
  ROOut3/1 -> Data Type Conversion2/1
  MinMax3/1 -> Memory3/1, MinMax/3
  [out2] -> ROOut2/2
  In2/1 -> ROOut2/1
  In3/1 -> ROOut3/1
  [out3] -> ROOut3/2
  MinMax/1 -> Out1/1
  Constant1/1 -> MinMax/1

== system c00006M_harness/Eval189 ==
  In2 : Inport
  In3 : Inport  Port=2
  Constant1 : Constant
  Data Type Conversion1 : DataTypeConversion
  Data Type Conversion2 : DataTypeConversion
  Memory2 : Memory  InitialCondition=1
  Memory3 : Memory  InitialCondition=1
  MinMax : MinMax  Inputs=3
  MinMax2 : MinMax  Inputs=2
  MinMax3 : MinMax  Inputs=2
  ROOut2 : RelationalOperator  Operator===  OutDataTypeStr=boolean  RndMeth=Simplest
  ROOut3 : RelationalOperator  Operator===  OutDataTypeStr=boolean  RndMeth=Simplest
  Out1 : Outport
  wires:
  Data Type Conversion2/1 -> MinMax3/1
  Data Type Conversion1/1 -> MinMax2/1
  MinMax2/1 -> MinMax/2, Memory2/1
  Memory2/1 -> MinMax2/2
  Memory3/1 -> MinMax3/2
  ROOut2/1 -> Data Type Conversion1/1
  ROOut3/1 -> Data Type Conversion2/1
  MinMax3/1 -> Memory3/1, MinMax/3
  [out2] -> ROOut2/2
  In2/1 -> ROOut2/1
  In3/1 -> ROOut3/1
  [out3] -> ROOut3/2
  MinMax/1 -> Out1/1
  Constant1/1 -> MinMax/1

== system c00006M_harness/Eval190 ==
  In2 : Inport
  In3 : Inport  Port=2
  Constant1 : Constant
  Data Type Conversion1 : DataTypeConversion
  Data Type Conversion2 : DataTypeConversion
  Memory2 : Memory  InitialCondition=1
  Memory3 : Memory  InitialCondition=1
  MinMax : MinMax  Inputs=3
  MinMax2 : MinMax  Inputs=2
  MinMax3 : MinMax  Inputs=2
  ROOut2 : RelationalOperator  Operator===  OutDataTypeStr=boolean  RndMeth=Simplest
  ROOut3 : RelationalOperator  Operator===  OutDataTypeStr=boolean  RndMeth=Simplest
  Out1 : Outport
  wires:
  Data Type Conversion2/1 -> MinMax3/1
  Data Type Conversion1/1 -> MinMax2/1
  MinMax2/1 -> MinMax/2, Memory2/1
  Memory2/1 -> MinMax2/2
  Memory3/1 -> MinMax3/2
  ROOut2/1 -> Data Type Conversion1/1
  ROOut3/1 -> Data Type Conversion2/1
  MinMax3/1 -> Memory3/1, MinMax/3
  [out2] -> ROOut2/2
  In2/1 -> ROOut2/1
  In3/1 -> ROOut3/1
  [out3] -> ROOut3/2
  MinMax/1 -> Out1/1
  Constant1/1 -> MinMax/1

== system c00006M_harness/Eval191 ==
  In2 : Inport
  In3 : Inport  Port=2
  Constant1 : Constant
  Data Type Conversion1 : DataTypeConversion
  Data Type Conversion2 : DataTypeConversion
  Memory2 : Memory  InitialCondition=1
  Memory3 : Memory  InitialCondition=1
  MinMax : MinMax  Inputs=3
  MinMax2 : MinMax  Inputs=2
  MinMax3 : MinMax  Inputs=2
  ROOut2 : RelationalOperator  Operator===  OutDataTypeStr=boolean  RndMeth=Simplest
  ROOut3 : RelationalOperator  Operator===  OutDataTypeStr=boolean  RndMeth=Simplest
  Out1 : Outport
  wires:
  Data Type Conversion2/1 -> MinMax3/1
  Data Type Conversion1/1 -> MinMax2/1
  MinMax2/1 -> MinMax/2, Memory2/1
  Memory2/1 -> MinMax2/2
  Memory3/1 -> MinMax3/2
  ROOut2/1 -> Data Type Conversion1/1
  ROOut3/1 -> Data Type Conversion2/1
  MinMax3/1 -> Memory3/1, MinMax/3
  [out2] -> ROOut2/2
  In2/1 -> ROOut2/1
  In3/1 -> ROOut3/1
  [out3] -> ROOut3/2
  MinMax/1 -> Out1/1
  Constant1/1 -> MinMax/1

== system c00006M_harness/Eval192 ==
  In2 : Inport
  In3 : Inport  Port=2
  Constant1 : Constant
  Data Type Conversion1 : DataTypeConversion
  Data Type Conversion2 : DataTypeConversion
  Memory2 : Memory  InitialCondition=1
  Memory3 : Memory  InitialCondition=1
  MinMax : MinMax  Inputs=3
  MinMax2 : MinMax  Inputs=2
  MinMax3 : MinMax  Inputs=2
  ROOut2 : RelationalOperator  Operator===  OutDataTypeStr=boolean  RndMeth=Simplest
  ROOut3 : RelationalOperator  Operator===  OutDataTypeStr=boolean  RndMeth=Simplest
  Out1 : Outport
  wires:
  Data Type Conversion2/1 -> MinMax3/1
  Data Type Conversion1/1 -> MinMax2/1
  MinMax2/1 -> MinMax/2, Memory2/1
  Memory2/1 -> MinMax2/2
  Memory3/1 -> MinMax3/2
  ROOut2/1 -> Data Type Conversion1/1
  ROOut3/1 -> Data Type Conversion2/1
  MinMax3/1 -> Memory3/1, MinMax/3
  [out2] -> ROOut2/2
  In2/1 -> ROOut2/1
  In3/1 -> ROOut3/1
  [out3] -> ROOut3/2
  MinMax/1 -> Out1/1
  Constant1/1 -> MinMax/1

== system c00006M_harness/Eval193 ==
  In2 : Inport
  In3 : Inport  Port=2
  Constant1 : Constant
  Data Type Conversion1 : DataTypeConversion
  Data Type Conversion2 : DataTypeConversion
  Memory2 : Memory  InitialCondition=1
  Memory3 : Memory  InitialCondition=1
  MinMax : MinMax  Inputs=3
  MinMax2 : MinMax  Inputs=2
  MinMax3 : MinMax  Inputs=2
  ROOut2 : RelationalOperator  Operator===  OutDataTypeStr=boolean  RndMeth=Simplest
  ROOut3 : RelationalOperator  Operator===  OutDataTypeStr=boolean  RndMeth=Simplest
  Out1 : Outport
  wires:
  Data Type Conversion2/1 -> MinMax3/1
  Data Type Conversion1/1 -> MinMax2/1
  MinMax2/1 -> MinMax/2, Memory2/1
  Memory2/1 -> MinMax2/2
  Memory3/1 -> MinMax3/2
  ROOut2/1 -> Data Type Conversion1/1
  ROOut3/1 -> Data Type Conversion2/1
  MinMax3/1 -> Memory3/1, MinMax/3
  [out2] -> ROOut2/2
  In2/1 -> ROOut2/1
  In3/1 -> ROOut3/1
  [out3] -> ROOut3/2
  MinMax/1 -> Out1/1
  Constant1/1 -> MinMax/1

== system c00006M_harness/Eval194 ==
  In2 : Inport
  In3 : Inport  Port=2
  Constant1 : Constant
  Data Type Conversion1 : DataTypeConversion
  Data Type Conversion2 : DataTypeConversion
  Memory2 : Memory  InitialCondition=1
  Memory3 : Memory  InitialCondition=1
  MinMax : MinMax  Inputs=3
  MinMax2 : MinMax  Inputs=2
  MinMax3 : MinMax  Inputs=2
  ROOut2 : RelationalOperator  Operator===  OutDataTypeStr=boolean  RndMeth=Simplest
  ROOut3 : RelationalOperator  Operator===  OutDataTypeStr=boolean  RndMeth=Simplest
  Out1 : Outport
  wires:
  Data Type Conversion2/1 -> MinMax3/1
  Data Type Conversion1/1 -> MinMax2/1
  MinMax2/1 -> MinMax/2, Memory2/1
  Memory2/1 -> MinMax2/2
  Memory3/1 -> MinMax3/2
  ROOut2/1 -> Data Type Conversion1/1
  ROOut3/1 -> Data Type Conversion2/1
  MinMax3/1 -> Memory3/1, MinMax/3
  [out2] -> ROOut2/2
  In2/1 -> ROOut2/1
  In3/1 -> ROOut3/1
  [out3] -> ROOut3/2
  MinMax/1 -> Out1/1
  Constant1/1 -> MinMax/1

== system c00006M_harness/Eval195 ==
  In2 : Inport
  In3 : Inport  Port=2
  Constant1 : Constant
  Data Type Conversion1 : DataTypeConversion
  Data Type Conversion2 : DataTypeConversion
  Memory2 : Memory  InitialCondition=1
  Memory3 : Memory  InitialCondition=1
  MinMax : MinMax  Inputs=3
  MinMax2 : MinMax  Inputs=2
  MinMax3 : MinMax  Inputs=2
  ROOut2 : RelationalOperator  Operator===  OutDataTypeStr=boolean  RndMeth=Simplest
  ROOut3 : RelationalOperator  Operator===  OutDataTypeStr=boolean  RndMeth=Simplest
  Out1 : Outport
  wires:
  Data Type Conversion2/1 -> MinMax3/1
  Data Type Conversion1/1 -> MinMax2/1
  MinMax2/1 -> MinMax/2, Memory2/1
  Memory2/1 -> MinMax2/2
  Memory3/1 -> MinMax3/2
  ROOut2/1 -> Data Type Conversion1/1
  ROOut3/1 -> Data Type Conversion2/1
  MinMax3/1 -> Memory3/1, MinMax/3
  [out2] -> ROOut2/2
  In2/1 -> ROOut2/1
  In3/1 -> ROOut3/1
  [out3] -> ROOut3/2
  MinMax/1 -> Out1/1
  Constant1/1 -> MinMax/1

== system c00006M_harness/Eval196 ==
  In2 : Inport
  In3 : Inport  Port=2
  Constant1 : Constant
  Data Type Conversion1 : DataTypeConversion
  Data Type Conversion2 : DataTypeConversion
  Memory2 : Memory  InitialCondition=1
  Memory3 : Memory  InitialCondition=1
  MinMax : MinMax  Inputs=3
  MinMax2 : MinMax  Inputs=2
  MinMax3 : MinMax  Inputs=2
  ROOut2 : RelationalOperator  Operator===  OutDataTypeStr=boolean  RndMeth=Simplest
  ROOut3 : RelationalOperator  Operator===  OutDataTypeStr=boolean  RndMeth=Simplest
  Out1 : Outport
  wires:
  Data Type Conversion2/1 -> MinMax3/1
  Data Type Conversion1/1 -> MinMax2/1
  MinMax2/1 -> MinMax/2, Memory2/1
  Memory2/1 -> MinMax2/2
  Memory3/1 -> MinMax3/2
  ROOut2/1 -> Data Type Conversion1/1
  ROOut3/1 -> Data Type Conversion2/1
  MinMax3/1 -> Memory3/1, MinMax/3
  [out2] -> ROOut2/2
  In2/1 -> ROOut2/1
  In3/1 -> ROOut3/1
  [out3] -> ROOut3/2
  MinMax/1 -> Out1/1
  Constant1/1 -> MinMax/1

== system c00006M_harness/Eval197 ==
  In2 : Inport
  In3 : Inport  Port=2
  Constant1 : Constant
  Data Type Conversion1 : DataTypeConversion
  Data Type Conversion2 : DataTypeConversion
  Memory2 : Memory  InitialCondition=1
  Memory3 : Memory  InitialCondition=1
  MinMax : MinMax  Inputs=3
  MinMax2 : MinMax  Inputs=2
  MinMax3 : MinMax  Inputs=2
  ROOut2 : RelationalOperator  Operator===  OutDataTypeStr=boolean  RndMeth=Simplest
  ROOut3 : RelationalOperator  Operator===  OutDataTypeStr=boolean  RndMeth=Simplest
  Out1 : Outport
  wires:
  Data Type Conversion2/1 -> MinMax3/1
  Data Type Conversion1/1 -> MinMax2/1
  MinMax2/1 -> MinMax/2, Memory2/1
  Memory2/1 -> MinMax2/2
  Memory3/1 -> MinMax3/2
  ROOut2/1 -> Data Type Conversion1/1
  ROOut3/1 -> Data Type Conversion2/1
  MinMax3/1 -> Memory3/1, MinMax/3
  [out2] -> ROOut2/2
  In2/1 -> ROOut2/1
  In3/1 -> ROOut3/1
  [out3] -> ROOut3/2
  MinMax/1 -> Out1/1
  Constant1/1 -> MinMax/1

== system c00006M_harness/Eval198 ==
  In2 : Inport
  In3 : Inport  Port=2
  Constant1 : Constant
  Data Type Conversion1 : DataTypeConversion
  Data Type Conversion2 : DataTypeConversion
  Memory2 : Memory  InitialCondition=1
  Memory3 : Memory  InitialCondition=1
  MinMax : MinMax  Inputs=3
  MinMax2 : MinMax  Inputs=2
  MinMax3 : MinMax  Inputs=2
  ROOut2 : RelationalOperator  Operator===  OutDataTypeStr=boolean  RndMeth=Simplest
  ROOut3 : RelationalOperator  Operator===  OutDataTypeStr=boolean  RndMeth=Simplest
  Out1 : Outport
  wires:
  Data Type Conversion2/1 -> MinMax3/1
  Data Type Conversion1/1 -> MinMax2/1
  MinMax2/1 -> MinMax/2, Memory2/1
  Memory2/1 -> MinMax2/2
  Memory3/1 -> MinMax3/2
  ROOut2/1 -> Data Type Conversion1/1
  ROOut3/1 -> Data Type Conversion2/1
  MinMax3/1 -> Memory3/1, MinMax/3
  [out2] -> ROOut2/2
  In2/1 -> ROOut2/1
  In3/1 -> ROOut3/1
  [out3] -> ROOut3/2
  MinMax/1 -> Out1/1
  Constant1/1 -> MinMax/1

== system c00006M_harness/Eval199 ==
  In2 : Inport
  In3 : Inport  Port=2
  Constant1 : Constant
  Data Type Conversion1 : DataTypeConversion
  Data Type Conversion2 : DataTypeConversion
  Memory2 : Memory  InitialCondition=1
  Memory3 : Memory  InitialCondition=1
  MinMax : MinMax  Inputs=3
  MinMax2 : MinMax  Inputs=2
  MinMax3 : MinMax  Inputs=2
  ROOut2 : RelationalOperator  Operator===  OutDataTypeStr=boolean  RndMeth=Simplest
  ROOut3 : RelationalOperator  Operator===  OutDataTypeStr=boolean  RndMeth=Simplest
  Out1 : Outport
  wires:
  Data Type Conversion2/1 -> MinMax3/1
  Data Type Conversion1/1 -> MinMax2/1
  MinMax2/1 -> MinMax/2, Memory2/1
  Memory2/1 -> MinMax2/2
  Memory3/1 -> MinMax3/2
  ROOut2/1 -> Data Type Conversion1/1
  ROOut3/1 -> Data Type Conversion2/1
  MinMax3/1 -> Memory3/1, MinMax/3
  [out2] -> ROOut2/2
  In2/1 -> ROOut2/1
  In3/1 -> ROOut3/1
  [out3] -> ROOut3/2
  MinMax/1 -> Out1/1
  Constant1/1 -> MinMax/1

== system c00006M_harness/Eval200 ==
  In2 : Inport
  In3 : Inport  Port=2
  Constant1 : Constant
  Data Type Conversion1 : DataTypeConversion
  Data Type Conversion2 : DataTypeConversion
  Memory2 : Memory  InitialCondition=1
  Memory3 : Memory  InitialCondition=1
  MinMax : MinMax  Inputs=3
  MinMax2 : MinMax  Inputs=2
  MinMax3 : MinMax  Inputs=2
  ROOut2 : RelationalOperator  Operator===  OutDataTypeStr=boolean  RndMeth=Simplest
  ROOut3 : RelationalOperator  Operator===  OutDataTypeStr=boolean  RndMeth=Simplest
  Out1 : Outport
  wires:
  Data Type Conversion2/1 -> MinMax3/1
  Data Type Conversion1/1 -> MinMax2/1
  MinMax2/1 -> MinMax/2, Memory2/1
  Memory2/1 -> MinMax2/2
  Memory3/1 -> MinMax3/2
  ROOut2/1 -> Data Type Conversion1/1
  ROOut3/1 -> Data Type Conversion2/1
  MinMax3/1 -> Memory3/1, MinMax/3
  [out2] -> ROOut2/2
  In2/1 -> ROOut2/1
  In3/1 -> ROOut3/1
  [out3] -> ROOut3/2
  MinMax/1 -> Out1/1
  Constant1/1 -> MinMax/1

== system c00006M_harness/Eval201 ==
  In2 : Inport
  In3 : Inport  Port=2
  Constant1 : Constant
  Data Type Conversion1 : DataTypeConversion
  Data Type Conversion2 : DataTypeConversion
  Memory2 : Memory  InitialCondition=1
  Memory3 : Memory  InitialCondition=1
  MinMax : MinMax  Inputs=3
  MinMax2 : MinMax  Inputs=2
  MinMax3 : MinMax  Inputs=2
  ROOut2 : RelationalOperator  Operator===  OutDataTypeStr=boolean  RndMeth=Simplest
  ROOut3 : RelationalOperator  Operator===  OutDataTypeStr=boolean  RndMeth=Simplest
  Out1 : Outport
  wires:
  Data Type Conversion2/1 -> MinMax3/1
  Data Type Conversion1/1 -> MinMax2/1
  MinMax2/1 -> MinMax/2, Memory2/1
  Memory2/1 -> MinMax2/2
  Memory3/1 -> MinMax3/2
  ROOut2/1 -> Data Type Conversion1/1
  ROOut3/1 -> Data Type Conversion2/1
  MinMax3/1 -> Memory3/1, MinMax/3
  [out2] -> ROOut2/2
  In2/1 -> ROOut2/1
  In3/1 -> ROOut3/1
  [out3] -> ROOut3/2
  MinMax/1 -> Out1/1
  Constant1/1 -> MinMax/1
